simulink subsystem "dvigatel"  (R2023a)
settings: Solver=VariableStepAuto  StartTime=0.0  StopTime=10.0  RelTol=1e-3
model mask{J=7e-6, Cm=1.3, Cw=3.15, L=0.0015, R=8, Lob=0.013, b=0.001}
settings Model: Creator=diontep  LastModifiedBy=diontep

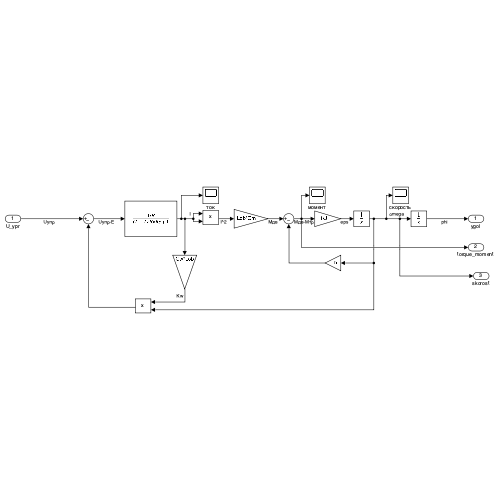
[thumbnail: Simulink's stored preview of the top-level diagram]
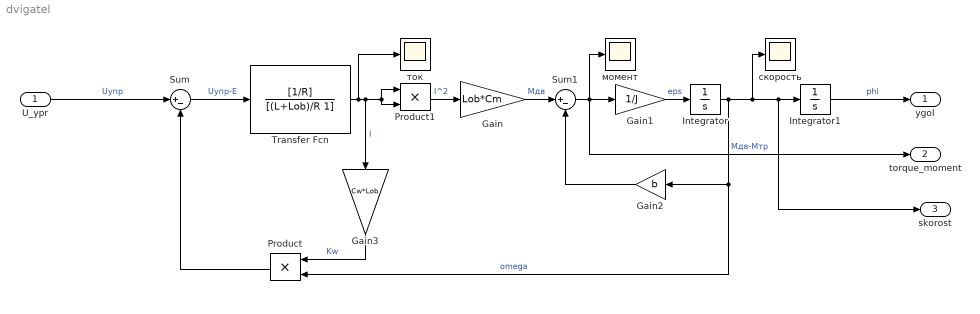
== system dvigatel ==
  U_ypr : Inport
  Gain : Gain  Gain=Lob*Cm
  Gain1 : Gain  Gain=1/J
  Gain2 : Gain  Gain=b
  Gain3 : Gain  Gain=Cw*Lob
  Integrator : Integrator
  Integrator1 : Integrator
  Product : Product
  Product1 : Product
  Sum : Sum  Inputs=|+-
  Sum1 : Sum  Inputs=|+-
  Transfer Fcn : TransferFcn  Numerator=[1/R]  Denominator=[(L+Lob)/R 1]
  момент : Scope
  скорость : Scope
  ток : Scope
  ygol : Outport
  torque_moment : Outport  Port=2
  skorost : Outport  Port=3
  wires:
  U_ypr/1 -> Sum/1  "Uупр"
  Gain1/1 -> Integrator/1  "eps"
  Sum/1 -> Transfer Fcn/1  "Uупр-E"
  Product1/1 -> Gain/1  "I^2"
  Transfer Fcn/1 -> ток/1, Product1/2, Product1/1, Gain3/1  "I"
  Product/1 -> Sum/2
  Integrator/1 -> skorost/1, Integrator1/1, скорость/1, Gain2/1, Product/2  "omega"
  Gain3/1 -> Product/1  "Kw"
  Gain/1 -> Sum1/1  "Mдв"
  Sum1/1 -> torque_moment/1, момент/1, Gain1/1  "Мдв-Мтр"
  Integrator1/1 -> ygol/1  "phi"
  Gain2/1 -> Sum1/2
